simulink model "rtwdemo_foreachreuse"  (Simulink 7.6)
settings: Solver=FixedStepDiscrete  StartTime=0.0  StopTime=10.0  RelTol=1e-3
libraries: rtwdemowidgets x1
Description:
  | Reusing Functions with Different Input Sizes
  | 
  | In this demo we illustrate the code reuse that happens when different For
  | Each Subsystems containing identically connected components are
  | fed with signals of different size.
settings Model: Creator=The MathWorks Inc.
settings DataIOCC: SaveFormat=Structure  SaveOutput=off  SaveTime=off
settings OptimizationCC: InlineParams=on  InlineInvariantSignals=on  StateBitsets=on  DataBitsets=on  UseTempVars=on  EfficientFloat2IntCast=on
settings HardwareCC: ProdBitPerLong=64  ProdIntDivRoundTo=Zero  ProdEndianess=LittleEndian  ProdWordSize=64  ProdHWDeviceType=Specified
settings RTWCC: GenerateReport=on  RTWVerbose=off  ProcessScript=grt_make_rtw_hook  LaunchReport=on
settings CodeAppCC: ForceParamTrailComments=on

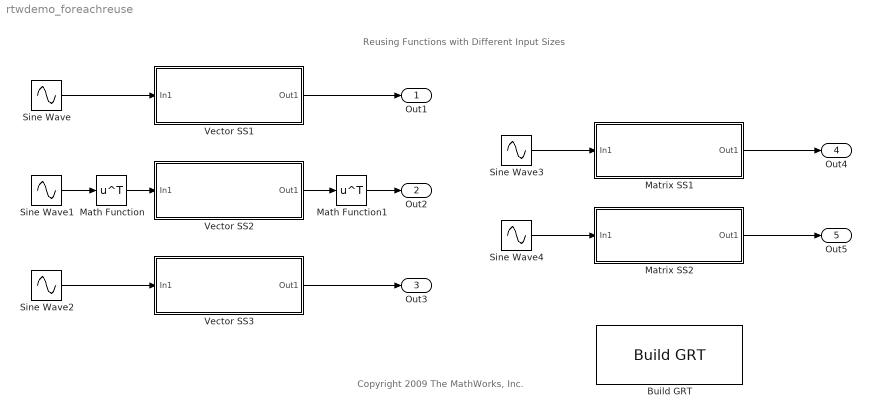
== system rtwdemo_foreachreuse ==
  note: Copyright 2009 The MathWorks, Inc.
  note: Reusing Functions with Different Input Sizes
  Build GRT : rtwdemowidgets/Build GRT  SystemSampleTime=-1  attrib_overrides={}
  Math Function : Math  Operator=transpose  SaturateOnIntegerOverflow=on
  Math Function1 : Math  Operator=transpose  SaturateOnIntegerOverflow=on
  Matrix SS1 : Subsystem  TreatAsAtomicUnit=on  RTWFcnName=MatrixProcessing
      settings: RTWFcnNameOpts=User specified  RTWFileNameOpts=Use function name
  Matrix SS2 : Subsystem  TreatAsAtomicUnit=on  RTWFcnName=MatrixProcessing
      settings: RTWFcnNameOpts=User specified  RTWFileNameOpts=Use function name
  Sine Wave : Sin  Amplitude=[1:10]'  SampleTime=.1  VectorParams1D=off
  Sine Wave1 : Sin  Amplitude=1:8  SampleTime=.1  VectorParams1D=off
  Sine Wave2 : Sin  Amplitude=1:7  SampleTime=.1
  Sine Wave3 : Sin  Amplitude=kron([1 1],eye(4))  SampleTime=.1  VectorParams1D=off
  Sine Wave4 : Sin  Amplitude=kron([1 1 1],eye(4))  SampleTime=.1  VectorParams1D=off
  Vector SS1 : Subsystem  TreatAsAtomicUnit=on  RTWFcnName=VectorProcessing
      settings: RTWFcnNameOpts=User specified  RTWFileNameOpts=Use function name
  Vector SS2 : Subsystem  TreatAsAtomicUnit=on  RTWFcnName=VectorProcessing
      settings: RTWFcnNameOpts=User specified  RTWFileNameOpts=Use function name
  Vector SS3 : Subsystem  TreatAsAtomicUnit=on  RTWFcnName=VectorProcessing
      settings: RTWFcnNameOpts=User specified  RTWFileNameOpts=Use function name
  Out1 : Outport
  Out2 : Outport  Port=2
  Out3 : Outport  Port=3
  Out4 : Outport  Port=4
  Out5 : Outport  Port=5
  wires:
  Sine Wave2/1 -> Vector SS3/1(In1)
  Vector SS3/1(Out1) -> Out3/1
  Sine Wave1/1 -> Math Function/1
  Vector SS2/1(Out1) -> Math Function1/1
  Math Function/1 -> Vector SS2/1(In1)
  Math Function1/1 -> Out2/1
  Vector SS1/1(Out1) -> Out1/1
  Sine Wave/1 -> Vector SS1/1(In1)
  Sine Wave3/1 -> Matrix SS1/1(In1)
  Matrix SS1/1(Out1) -> Out4/1
  Sine Wave4/1 -> Matrix SS2/1(In1)
  Matrix SS2/1(Out1) -> Out5/1

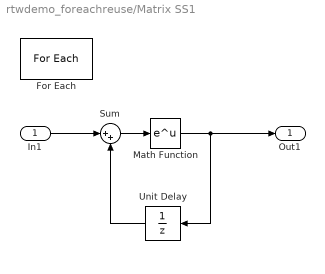
== system rtwdemo_foreachreuse/Matrix SS1 ==
  In1 : Inport  Partition=on  PartitionDimension=2  PartitionWidth=4
  For Each : ForEach  IndexMode=One-based
  Math Function : Math  SaturateOnIntegerOverflow=on
  Sum : Sum  Inputs=|++
  Unit Delay : UnitDelay  SampleTime=-1
  Out1 : Outport  ConcatenationDimension=2
  wires:
  Sum/1 -> Math Function/1
  Unit Delay/1 -> Sum/2
  Math Function/1 -> Out1/1, Unit Delay/1
  In1/1 -> Sum/1

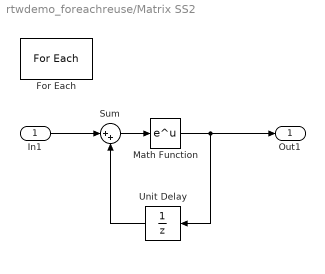
== system rtwdemo_foreachreuse/Matrix SS2 ==
  In1 : Inport  Partition=on  PartitionDimension=2  PartitionWidth=4
  For Each : ForEach  IndexMode=One-based
  Math Function : Math  SaturateOnIntegerOverflow=on
  Sum : Sum  Inputs=|++
  Unit Delay : UnitDelay  SampleTime=-1
  Out1 : Outport  ConcatenationDimension=2
  wires:
  In1/1 -> Sum/1
  Math Function/1 -> Unit Delay/1, Out1/1
  Unit Delay/1 -> Sum/2
  Sum/1 -> Math Function/1

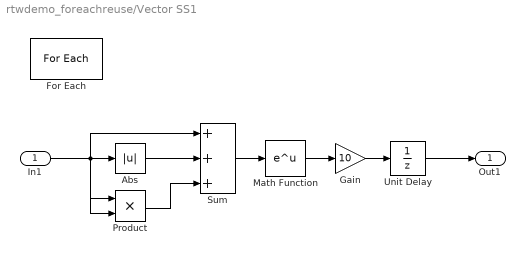
== system rtwdemo_foreachreuse/Vector SS1 ==
  In1 : Inport  Partition=on  PartitionDimension=1  PartitionWidth=1
  Abs : Abs
  For Each : ForEach  IndexMode=One-based
  Gain : Gain  Gain=10
  Math Function : Math  SaturateOnIntegerOverflow=on
  Product : Product  RndMeth=Zero
  Sum : Sum  Inputs=3
  Unit Delay : UnitDelay  SampleTime=-1
  Out1 : Outport  ConcatenationDimension=1
  wires:
  Gain/1 -> Unit Delay/1
  Abs/1 -> Sum/2
  Product/1 -> Sum/3
  Sum/1 -> Math Function/1
  Math Function/1 -> Gain/1
  Unit Delay/1 -> Out1/1
  In1/1 -> Sum/1, Abs/1, Product/1, Product/2

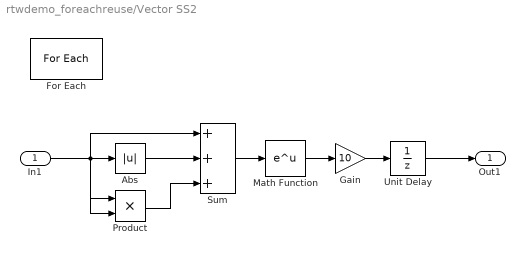
== system rtwdemo_foreachreuse/Vector SS2 ==
  In1 : Inport  Partition=on  PartitionDimension=1  PartitionWidth=1
  Abs : Abs
  For Each : ForEach  IndexMode=One-based
  Gain : Gain  Gain=10
  Math Function : Math  SaturateOnIntegerOverflow=on
  Product : Product  RndMeth=Zero
  Sum : Sum  Inputs=3
  Unit Delay : UnitDelay  SampleTime=-1
  Out1 : Outport  ConcatenationDimension=1
  wires:
  In1/1 -> Product/2, Product/1, Abs/1, Sum/1
  Unit Delay/1 -> Out1/1
  Math Function/1 -> Gain/1
  Sum/1 -> Math Function/1
  Product/1 -> Sum/3
  Abs/1 -> Sum/2
  Gain/1 -> Unit Delay/1

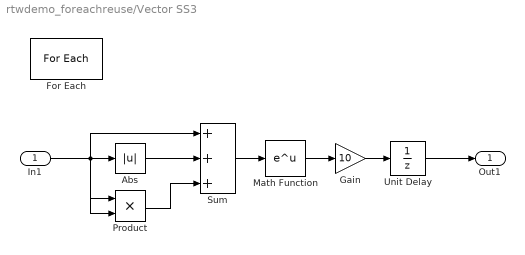
== system rtwdemo_foreachreuse/Vector SS3 ==
  In1 : Inport  Partition=on  PartitionDimension=1  PartitionWidth=1
  Abs : Abs
  For Each : ForEach  IndexMode=One-based
  Gain : Gain  Gain=10
  Math Function : Math  SaturateOnIntegerOverflow=on
  Product : Product  RndMeth=Zero
  Sum : Sum  Inputs=3
  Unit Delay : UnitDelay  SampleTime=-1
  Out1 : Outport  ConcatenationDimension=1
  wires:
  Gain/1 -> Unit Delay/1
  Abs/1 -> Sum/2
  Product/1 -> Sum/3
  Sum/1 -> Math Function/1
  Math Function/1 -> Gain/1
  Unit Delay/1 -> Out1/1
  In1/1 -> Sum/1, Abs/1, Product/1, Product/2
